simulink model "keyboard_test"  (Simulink 7.6)
settings: Solver=ode45  StartTime=0.0  StopTime=inf  FixedStep=0.05  RelTol=1e-3
libraries: realtime_pacer_lib x1
settings Model: Creator=Nikola  LastModifiedBy=Nikola

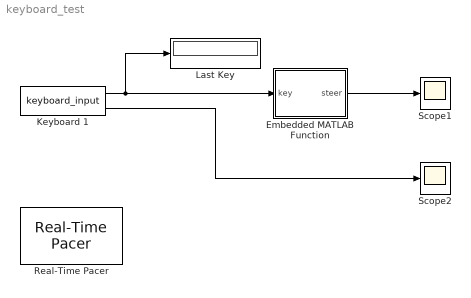
== system keyboard_test ==
  Embedded MATLAB Function : Stateflow chart  TreatAsAtomicUnit=on
  Keyboard 1 : M-S-Function  FunctionName=keyboard_input
      mask Type: Keyboard Input
      mask Description: Keyboard Input
      mask Display: fprintf('Keyboard');
  Last Key : Display
  Real-Time Pacer : realtime_pacer_lib/Real-Time Pacer  simTimePerRealTime=1
  Scope1 : Scope
      settings: YMin=0  YMax=250
  Scope2 : Scope
      settings: YMin=0  YMax=250
  wires:
  Keyboard 1/1 -> Last Key/1, Embedded MATLAB Function/1(key)
  Embedded MATLAB Function/1(steer) -> Scope1/1
  Keyboard 1/2 -> Scope2/1

== matlab function Embedded MATLAB Function ==
  data: key input double; steer output double
function steer = fcn(key)
%#eml

if(key==29)
    steer = 240;
elseif(key==28)
    steer = 0;
else
    steer = 120;
end
